simulink model "UkladNieZeroweWarunki"  (R2016a)
settings: Solver=ode45  StartTime=0.0  StopTime=10.0  MinStep=0.001  RelTol=1e-5
values from neighbouring files (symbols this model uses):
  A = [-100 0 0 ... (first row only)    [zad1.m]
  B = [1000 ... (first row only)    [zad1.m]
  C = [0 0 0.4]    [zad1.m]
  G = [-990720; 10957.5; -77.5]    [zad1.m]
settings Model: Creator=student  LastModifiedBy=student

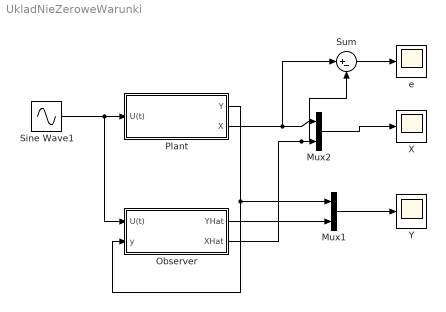
== system UkladNieZeroweWarunki ==
  Mux1 : Mux  Inputs=2
  Mux2 : Mux  Inputs=2
  "Observer " : Subsystem
  Plant : Subsystem
  Sine Wave1 : Sin  SampleTime=0
  Sum : Sum  Inputs=|+-
  X : Scope
  Y : Scope
  e : Scope
  wires:
  Sine Wave1/1 -> "Observer "/1(U(t)), Plant/1(U(t))
  Plant/1(Y) -> Mux1/1, "Observer "/2("y ")
  "Observer "/1(YHat) -> Mux1/2
  Plant/2(X) -> Sum/1, Mux2/1
  "Observer "/2(XHat) -> Sum/2, Mux2/2
  Mux2/1 -> X/1
  Mux1/1 -> Y/1
  Sum/1 -> e/1

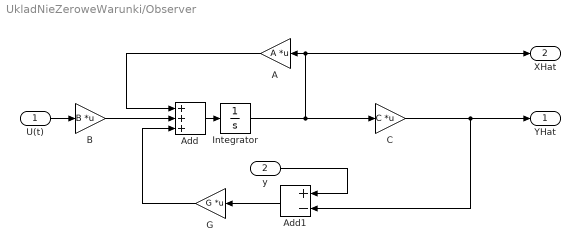
== system UkladNieZeroweWarunki/Observer  ==
  U(t) : Inport
  "y " : Inport  Port=2
  A : Gain  Gain=A  Multiplication=Matrix(K*u)
  Add : Sum  Inputs=+++
  Add1 : Sum  Inputs=+-
  B : Gain  Gain=B  Multiplication=Matrix(K*u)
  C : Gain  Gain=C  Multiplication=Matrix(K*u)
  G : Gain  Gain=G  Multiplication=Matrix(K*u)
  Integrator : Integrator  InitialCondition=[1 1 1]
  YHat : Outport
  XHat : Outport  Port=2
  wires:
  A/1 -> Add/1
  U(t)/1 -> B/1
  Integrator/1 -> C/1, XHat/1, A/1
  C/1 -> Add1/2, YHat/1
  B/1 -> Add/2
  "y "/1 -> Add1/1
  Add1/1 -> G/1
  G/1 -> Add/3
  Add/1 -> Integrator/1

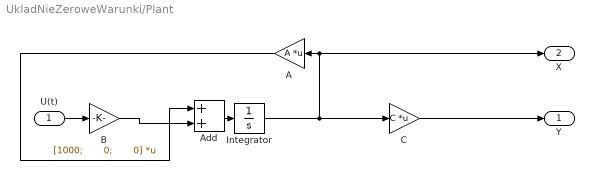
== system UkladNieZeroweWarunki/Plant ==
  U(t) : Inport
  A : Gain  Gain=A  Multiplication=Matrix(K*u)
  Add : Sum
  B : Gain  Gain=|  Multiplication=Matrix(K*u)
      | [1000;
      |       0;
      |       0]
  C : Gain  Gain=C  Multiplication=Matrix(K*u)
  Integrator : Integrator  InitialCondition=[0 0 0]
  Y : Outport
  X : Outport  Port=2
  wires:
  A/1 -> Add/1
  U(t)/1 -> B/1
  Integrator/1 -> C/1, X/1, A/1
  C/1 -> Y/1
  B/1 -> Add/2
  Add/1 -> Integrator/1
